simulink model "FCEvPowertrainController"  (R2024a)
settings: configuration reference "VehicleFixed10ms" (kept outside this file)
undefined symbols (not defined in the file): BattChrgMax, BattDischrgMax, ChrgLmt_bpt, CtrlBcuTrlrBrkGain, CtrlVcuEvChrgLmtBpt, CtrlVcuEvRegenBrkCutOff, CtrlVcuEvRegenBrkSpdBpt, CtrlVcuEvSocBpt, DischrgLmt_bpt, FCctrl, PlntBrkActrBoreFrnt, PlntBrkFrntBias, PlntBrkKinFricCffFrnt, PlntBrkNumPadsFrnt, PlntBrkPadMeanRadiusFrnt, PlntBrkPrsFctr, PlntBrkRearBias, PlntDiffrntlRatio, PlntEM1EffTbl, PlntEM1Spd, PlntEM1SpdEff, PlntEM1Trq, PlntEM1TrqEff, SOC_bpt
libraries: simulink x6, slpidlib x1, autolibutils x1
settings Model: DataDictionary=VirtualVehicleTemplate.sldd  ModifiedByFormat=The MathWorks, Inc.  SimulationMode=accelerator  Creator=The MathWorks, Inc.  LastModifiedBy=The MathWorks, Inc.
settings ConfigSetRef: SourceName=VehicleFixed10ms

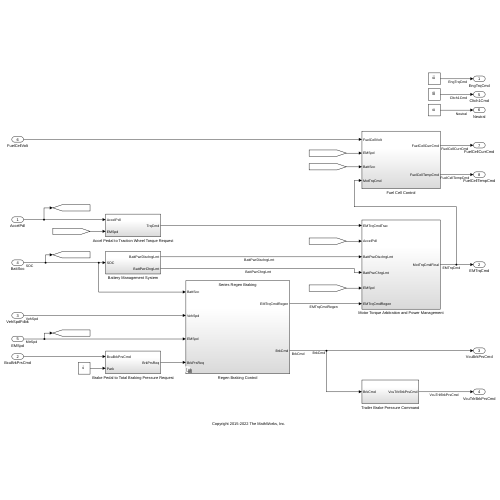
[thumbnail: Simulink's stored preview of the top-level diagram]
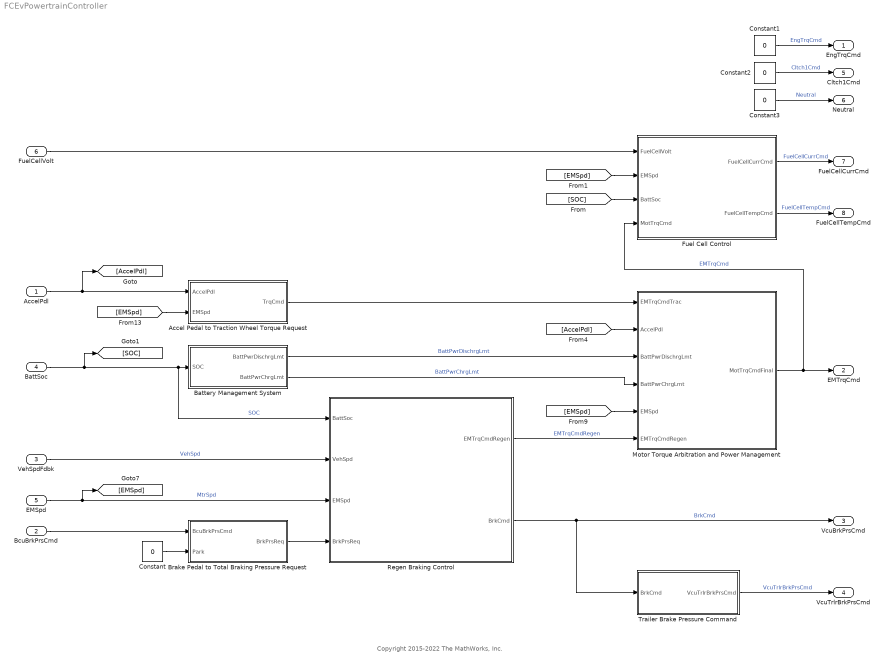
== system FCEvPowertrainController ==
  note: Copyright 2015-2022 The MathWorks, Inc.
  AccelPdl : Inport
  BcuBrkPrsCmd : Inport  Port=2  OutDataTypeStr=double  PortDimensions=4
  VehSpdFdbk : Inport  Port=3
  BattSoc : Inport  Port=4
  EMSpd : Inport  Port=5
  FuelCellVolt : Inport  Port=6
  Accel Pedal to Traction Wheel Torque Request : Subsystem  InitFcn=[~]=autosharedicon('autolibinternalvvblock',gcb,0);
  Battery Management System : Subsystem
  Brake Pedal to Total Braking Pressure Request : Subsystem
  Constant : Constant  Value=0
  Constant1 : Constant  Value=0  SampleTime=-1
  Constant2 : Constant  Value=0  SampleTime=-1
  Constant3 : Constant  Value=0  SampleTime=-1
  Fuel Cell Control : Subsystem
  Motor Torque Arbitration and Power Management : Subsystem
  Regen Braking Control : Subsystem  Variant=on  VariantControlMode=label  VariantControl=(default)  LabelModeActiveChoice=Variant
  Trailer Brake Pressure Command : Subsystem
  EngTrqCmd : Outport  OutDataTypeStr=double  PortDimensions=1  SampleTime=[0.01,0]  VectorParamsAs1DForOutWhenUnconnected=off
  EMTrqCmd : Outport  Port=2  VectorParamsAs1DForOutWhenUnconnected=off
  VcuBrkPrsCmd : Outport  Port=3  PortDimensions=4  VectorParamsAs1DForOutWhenUnconnected=off
  VcuTrlrBrkPrsCmd : Outport  Port=4  PortDimensions=6  VectorParamsAs1DForOutWhenUnconnected=off
  Cltch1Cmd : Outport  Port=5  PortDimensions=1  SampleTime=[0.01,0]  VectorParamsAs1DForOutWhenUnconnected=off
  Neutral : Outport  Port=6  PortDimensions=1  SampleTime=[0.01,0]  VectorParamsAs1DForOutWhenUnconnected=off
  FuelCellCurrCmd : Outport  Port=7  SampleTime=.01
  FuelCellTempCmd : Outport  Port=8
  wires:
  [AccelPdl] -> Motor Torque Arbitration and Power Management/2(AccelPdl)
  Battery Management System/1(BattPwrDischrgLmt) -> Motor Torque Arbitration and Power Management/3(BattPwrDischrgLmt)  "BattPwrDischrgLmt"
  BcuBrkPrsCmd/1 -> Brake Pedal to Total Braking Pressure Request/1(BcuBrkPrsCmd)
  Constant/1 -> Brake Pedal to Total Braking Pressure Request/2(Park)
  Battery Management System/2(BattPwrChrgLmt) -> Motor Torque Arbitration and Power Management/4("BattPwrChrgLmt ")  "BattPwrChrgLmt"
  Brake Pedal to Total Braking Pressure Request/1(BrkPrsReq) -> Regen Braking Control/4("BrkPrsReq ")
  [EMSpd] -> Accel Pedal to Traction Wheel Torque Request/2(EMSpd)
  VehSpdFdbk/1 -> Regen Braking Control/2("VehSpd ")  "VehSpd"
  BattSoc/1 -> [SOC], Regen Braking Control/1("BattSoc "), Battery Management System/1(SOC)  "SOC"
  Accel Pedal to Traction Wheel Torque Request/1(TrqCmd) -> Motor Torque Arbitration and Power Management/1(EMTrqCmdTrac)
  EMSpd/1 -> Regen Braking Control/3("EMSpd "), [EMSpd]  "MtrSpd"
  AccelPdl/1 -> [AccelPdl], Accel Pedal to Traction Wheel Torque Request/1(AccelPdl)
  [EMSpd] -> Motor Torque Arbitration and Power Management/5(EMSpd)
  Motor Torque Arbitration and Power Management/1(MotTrqCmdFinal) -> Fuel Cell Control/4(MotTrqCmd), EMTrqCmd/1  "EMTrqCmd"
  Regen Braking Control/1(" EMTrqCmdRegen") -> Motor Torque Arbitration and Power Management/6(EMTrqCmdRegen)  "EMTrqCmdRegen"
  FuelCellVolt/1 -> Fuel Cell Control/1(FuelCellVolt)
  [EMSpd] -> Fuel Cell Control/2(EMSpd)
  [SOC] -> Fuel Cell Control/3(BattSoc)
  Fuel Cell Control/1(FuelCellCurrCmd) -> FuelCellCurrCmd/1  "FuelCellCurrCmd"
  Fuel Cell Control/2(FuelCellTempCmd) -> FuelCellTempCmd/1  "FuelCellTempCmd"
  Constant3/1 -> Neutral/1  "Neutral"
  Constant2/1 -> Cltch1Cmd/1  "Cltch1Cmd"
  Constant1/1 -> EngTrqCmd/1  "EngTrqCmd"
  Trailer Brake Pressure Command/1(VcuTrlrBrkPrsCmd) -> VcuTrlrBrkPrsCmd/1  "VcuTrlrBrkPrsCmd"
  Regen Braking Control/2(" BrkCmd") -> Trailer Brake Pressure Command/1(BrkCmd), VcuBrkPrsCmd/1  "BrkCmd"

== system FCEvPowertrainController/Accel Pedal to Traction Wheel Torque Request ==
  note: Convert Accelerator Pedal Position to Torque Command
      | using Motor Torque Speed Curve
  AccelPdl : Inport
  EMSpd : Inport  Port=2
  MaxEMTrqVsSpd : Lookup_n-D  NumberOfTableDimensions=1  BreakpointsForDimension1=PlntEM1Spd  Table=PlntEM1Trq  ExtrapMethod=Clip  UseLastTableValue=on  InternalRulePriority=Speed  OutDataTypeStr=Inherit: Inherit from 'Table data'  RndMeth=Simplest
  Product1 : Product
  rads_to_rpm : Gain  Gain=30/pi
  TrqCmd : Outport  VectorParamsAs1DForOutWhenUnconnected=off
  wires:
  Product1/1 -> TrqCmd/1
  MaxEMTrqVsSpd/1 -> Product1/2
  AccelPdl/1 -> Product1/1
  EMSpd/1 -> rads_to_rpm/1
  rads_to_rpm/1 -> MaxEMTrqVsSpd/1

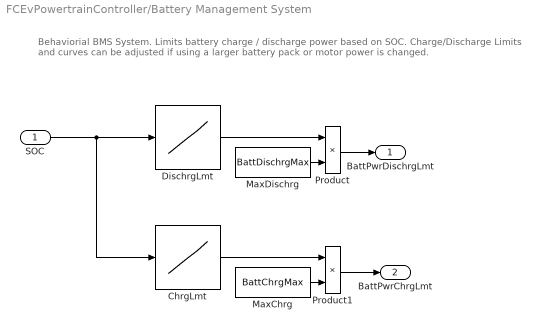
== system FCEvPowertrainController/Battery Management System ==
  note: Behaviorial BMS System. Limits battery charge / discharge power based on SOC.
      |
      | Charge/Discharge Limits and curves can be adjusted if using a larger battery pack
      | or motor power is changed.
  SOC : Inport
  ChrgLmt : Lookup_n-D  NumberOfTableDimensions=1  BreakpointsForDimension1=SOC_bpt  Table=ChrgLmt_bpt  ExtrapMethod=Clip  UseLastTableValue=on  InternalRulePriority=Speed  RndMeth=Simplest
  DischrgLmt : Lookup_n-D  NumberOfTableDimensions=1  BreakpointsForDimension1=SOC_bpt  Table=DischrgLmt_bpt  ExtrapMethod=Clip  UseLastTableValue=on  InternalRulePriority=Speed  RndMeth=Simplest
  MaxChrg : Constant  Value=BattChrgMax
  MaxDischrg : Constant  Value=BattDischrgMax
  Product : Product
  Product1 : Product
  BattPwrDischrgLmt : Outport  VectorParamsAs1DForOutWhenUnconnected=off
  BattPwrChrgLmt : Outport  Port=2  VectorParamsAs1DForOutWhenUnconnected=off
  wires:
  SOC/1 -> DischrgLmt/1, ChrgLmt/1
  MaxChrg/1 -> Product1/2
  MaxDischrg/1 -> Product/2
  Product/1 -> BattPwrDischrgLmt/1
  Product1/1 -> BattPwrChrgLmt/1
  ChrgLmt/1 -> Product1/1
  DischrgLmt/1 -> Product/1

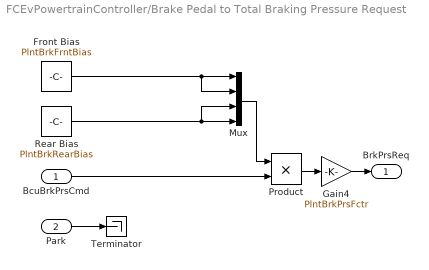
== system FCEvPowertrainController/Brake Pedal to Total Braking Pressure Request ==
  BcuBrkPrsCmd : Inport
  Park : Inport  Port=2
  Front Bias : Constant  Value=PlntBrkFrntBias
  Gain4 : Gain  Gain=PlntBrkPrsFctr
  Mux : Mux
  Product : Product
  Rear Bias : Constant  Value=PlntBrkRearBias
  Terminator : Terminator
  BrkPrsReq : Outport  VectorParamsAs1DForOutWhenUnconnected=off
  wires:
  BcuBrkPrsCmd/1 -> Product/2
  Mux/1 -> Product/1
  Rear Bias/1 -> Mux/4, Mux/3
  Front Bias/1 -> Mux/1, Mux/2
  Gain4/1 -> BrkPrsReq/1
  Product/1 -> Gain4/1
  Park/1 -> Terminator/1

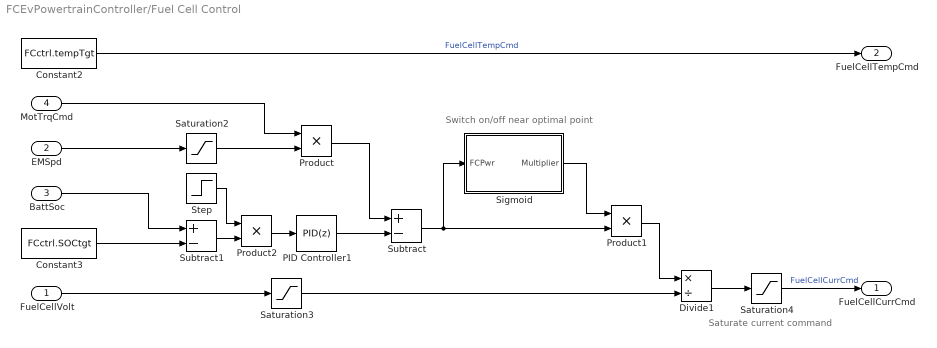
== system FCEvPowertrainController/Fuel Cell Control ==
  note: Switch on/off near optimal point
  note: Saturate current command
  FuelCellVolt : Inport
  EMSpd : Inport  Port=2
  BattSoc : Inport  Port=3
  MotTrqCmd : Inport  Port=4
  Constant2 : Constant  Value=FCctrl.tempTgt  SampleTime=0.01
  Constant3 : Constant  Value=FCctrl.SOCtgt
  Divide1 : Product  Inputs=*/
  PID Controller1 : slpidlib/PID Controller  Controller=PID  Form=Parallel  TimeDomain=Discrete-time  UseExternalTs=off  SampleTime=-1  IntegratorMethod=Forward Euler  FilterMethod=Forward Euler  ControllerParametersSource=internal  P=10000/2  I=0  UseKiTs=off  D=0  UseExternalDerivativeSource=off  N=100  UseFilter=on  TunerSelectOption=Transfer Function Based (PID Tuner App)  ZeroCross=off  InitialConditionSource=internal  InitialConditionForIntegrator=0  InitialConditionForFilter=0  DifferentiatorICPrevScaledInput=0  ExternalReset=none  TrackingMode=off  Kt=1  LimitOutput=off  SatLimitsSource=internal  UpperSaturationLimit=inf  LowerSaturationLimit=-inf  LinearizeAsGain=on  AntiWindupMode=none  Kb=1  LimitIntegrator=off  UpperIntegratorSaturationLimit=inf  LowerIntegratorSaturationLimit=-inf  POutMin=[]  POutMax=[]  IOutMin=[]  IOutMax=[]  DOutMin=[]  DOutMax=[]  NOutMin=[]  NOutMax=[]  SumOutMin=[]  SumOutMax=[]  SaturationOutMin=[]  SaturationOutMax=[]  PParamMin=[]  PParamMax=[]  IParamMin=[]  IParamMax=[]  DParamMin=[]  DParamMax=[]  NParamMin=[]  NParamMax=[]  KbParamMin=[]  KbParamMax=[]  KtParamMin=[]  KtParamMax=[]  KbOutMin=[]  KbOutMax=[]  KtOutMin=[]  KtOutMax=[]  IntegratorOutMin=[]  IntegratorOutMax=[]  FilterOutMin=[]  FilterOutMax=[]  SumI1OutMin=[]  SumI1OutMax=[]  SumI2OutMin=[]  SumI2OutMax=[]  SumI3OutMin=[]  SumI3OutMax=[]  SumI4OutMin=[]  SumI4OutMax=[]  SumDOutMin=[]  SumDOutMax=[]  DifferentiatorOutMin=[]  DifferentiatorOutMax=[]  FilterDiffOutCoefMin=[]  FilterDiffOutCoefMax=[]  ReciprocalOutMin=[]  ReciprocalOutMax=[]  SumDenOutMin=[]  SumDenOutMax=[]  SumNumOutMin=[]  SumNumOutMax=[]  DivideOutMin=[]  DivideOutMax=[]  UdiffTsProdOutMin=[]  UdiffTsProdOutMax=[]  NTsProdOutMin=[]  NTsProdOutMax=[]  UintegralTsProdOutMin=[]  UintegralTsProdOutMax=[]  UngainTsProdOutMin=[]  UngainTsProdOutMax=[]  ClampingZeroOutDataTypeStr=Inherit: Inherit via back propagation  ClampingZeroOutMin=[]  ClampingZeroOutMax=[]  FilterDenConstantOutDataTypeStr=Inherit: Inherit via back propagation  FilterDenConstantOutMin=[]  FilterDenConstantOutMax=[]  PCopyOutDataTypeStr=Inherit: Inherit via back propagation  PCopyOutMin=[]  PCopyOutMax=[]  NCopyOutDataTypeStr=Inherit: Inherit via back propagation  NCopyOutMin=[]  NCopyOutMax=[]  IntegratorContinuousStateAttributes=''  IntegratorStateMustResolveToSignalObject=off  IntegratorRTWStateStorageClass=Auto  FilterContinuousStateAttributes=''  FilterStateMustResolveToSignalObject=off  FilterRTWStateStorageClass=Auto  ParallelPVariant=InternalParameters  IdealPVariant=Disabled  IVariant=InternalParameters  DVariant=InternalParameters  IntegratorVariant=Discrete  SatVariant=Disabled  AWVariant=Passthrough  PCopyVariant=Disabled  TRVariant=Disabled  FdbkBlocksVariant=Forward  IdealPFdbkVariant=Disabled  SatFdbkVariant=Disabled  DerivativeFilterVariant=ForwardEulerFilter  NVariant=InternalParameters  NCopyVariant=Disabled  FilterICVariant=InternalICsFilter  IntegratorICVariant=InternalICs  ExternalResetVariant=Disabled  TRSumVariant=Passthrough  SumFdbkVariant=Disabled  SumVariant=Sum_PID  TsampFilterVariant=InternalTs  TsampNgainVariant=Passthrough  TsampIntegralVariant=Disabled_SignalSpec  ExternalSaturationOutDataTypeStr=Inherit: Same as second input  DerivativeSourceVariant=ErrorSignal
  Product : Product
  Product1 : Product
  Product2 : Product
  Saturation2 : Saturate  UpperLimit=inf  LowerLimit=1  ZeroCross=off
  Saturation3 : Saturate  UpperLimit=inf  LowerLimit=200  ZeroCross=off
  Saturation4 : Saturate  UpperLimit=350  LowerLimit=0  ZeroCross=off
  Sigmoid : Subsystem
  Step : Step  SampleTime=0.01
  Subtract : Sum  Inputs=+-
  Subtract1 : Sum  Inputs=+-
  FuelCellCurrCmd : Outport  SampleTime=.01
  FuelCellTempCmd : Outport  Port=2
  wires:
  MotTrqCmd/1 -> Product/1
  Saturation4/1 -> FuelCellCurrCmd/1  "FuelCellCurrCmd"
  PID Controller1/1 -> Subtract/2
  Sigmoid/1(Multiplier) -> Product1/1
  Divide1/1 -> Saturation4/1
  Saturation3/1 -> Divide1/2
  Subtract/1 -> Product1/2, Sigmoid/1(FCPwr)
  Product/1 -> Subtract/1
  EMSpd/1 -> Saturation2/1
  Saturation2/1 -> Product/2
  BattSoc/1 -> Subtract1/1
  FuelCellVolt/1 -> Saturation3/1
  Product1/1 -> Divide1/1
  Constant3/1 -> Subtract1/2
  Constant2/1 -> FuelCellTempCmd/1  "FuelCellTempCmd"
  Subtract1/1 -> Product2/2
  Product2/1 -> PID Controller1/1
  Step/1 -> Product2/1

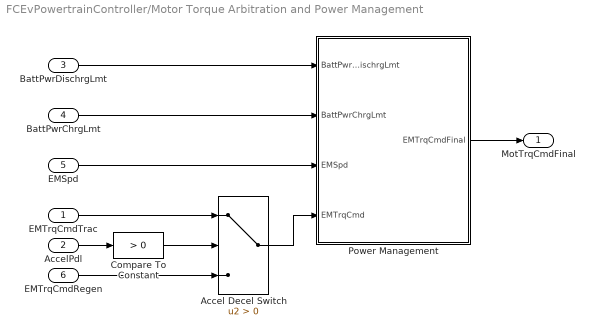
== system FCEvPowertrainController/Motor Torque Arbitration and Power Management ==
  EMTrqCmdTrac : Inport
  AccelPdl : Inport  Port=2
  BattPwrDischrgLmt : Inport  Port=3
  "BattPwrChrgLmt " : Inport  Port=4
  EMSpd : Inport  Port=5
  EMTrqCmdRegen : Inport  Port=6
  Accel Decel Switch : Switch  Criteria=u2 > Threshold  SaturateOnIntegerOverflow=off  InputSameDT=off
  Compare To Constant : simulink/Logic and Bit Operations/Compare To Constant  relop=>  const=0  OutDataTypeStr=boolean
  Power Management : Subsystem
  MotTrqCmdFinal : Outport  VectorParamsAs1DForOutWhenUnconnected=off
  wires:
  AccelPdl/1 -> Compare To Constant/1
  EMTrqCmdRegen/1 -> Accel Decel Switch/3
  EMTrqCmdTrac/1 -> Accel Decel Switch/1
  Power Management/1(EMTrqCmdFinal) -> MotTrqCmdFinal/1
  Accel Decel Switch/1 -> Power Management/4(EMTrqCmd)
  BattPwrDischrgLmt/1 -> Power Management/1(BattPwrDischrgLmt)
  "BattPwrChrgLmt "/1 -> Power Management/2(BattPwrChrgLmt)
  EMSpd/1 -> Power Management/3(EMSpd)
  Compare To Constant/1 -> Accel Decel Switch/2

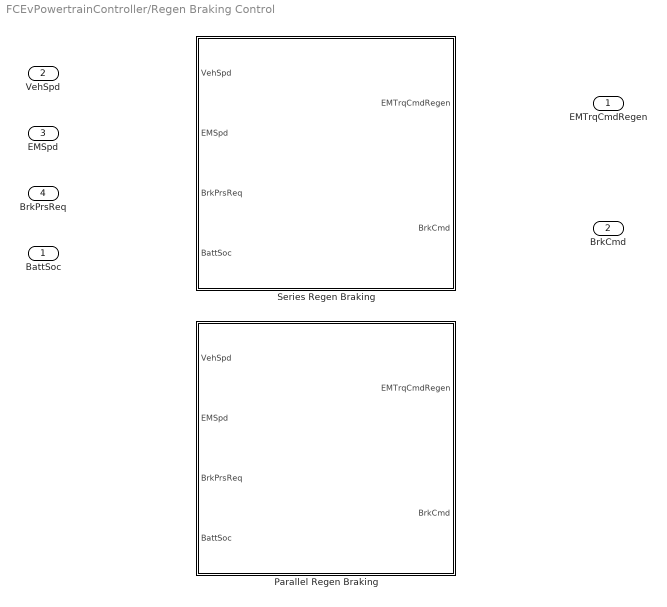
== system FCEvPowertrainController/Regen Braking Control ==
  "BattSoc " : Inport
  "VehSpd " : Inport  Port=2
  "EMSpd " : Inport  Port=3
  "BrkPrsReq " : Inport  Port=4
  Parallel Regen Braking : Subsystem  InitFcn=[~]=autosharedicon('autolibinternalvvblock',gcb,0);  VariantControl=(default)
  Series Regen Braking : Subsystem  InitFcn=[~]=autosharedicon('autolibinternalvvblock',gcb,0);  VariantControl=Variant
  " EMTrqCmdRegen" : Outport  VectorParamsAs1DForOutWhenUnconnected=off
  " BrkCmd" : Outport  Port=2  VectorParamsAs1DForOutWhenUnconnected=off

== system FCEvPowertrainController/Trailer Brake Pressure Command ==
  BrkCmd : Inport
  Gain1 : Gain  Gain=CtrlBcuTrlrBrkGain
  Probe : Probe  ProbeSampleTime=off  ProbeComplexSignal=off
  Product : Product  Inputs=*/
  Selector2 : Selector  InputPortWidth=1  IndexOptions=Index vector (dialog)  Indices=[1 1 1 1 1 1]  OutputSizes=1
  Sum : Sum  Inputs=+
  VcuTrlrBrkPrsCmd : Outport
  wires:
  Gain1/1 -> Selector2/1
  Product/1 -> Gain1/1
  Probe/1 -> Product/2
  BrkCmd/1 -> Probe/1, Sum/1
  Sum/1 -> Product/1
  Selector2/1 -> VcuTrlrBrkPrsCmd/1

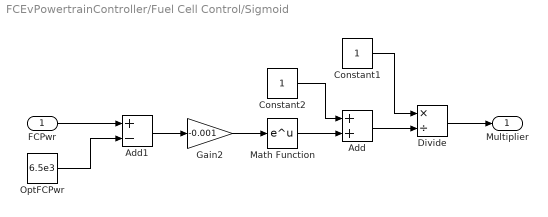
== system FCEvPowertrainController/Fuel Cell Control/Sigmoid ==
  FCPwr : Inport
  Add : Sum
  Add1 : Sum  Inputs=+-
  Constant1 : Constant
  Constant2 : Constant
  Divide : Product  Inputs=*/
  Gain2 : Gain  Gain=-0.001
  Math Function : Math
  OptFCPwr : Constant  Value=6.5e3
  Multiplier : Outport
  wires:
  Add1/1 -> Gain2/1
  Divide/1 -> Multiplier/1
  Math Function/1 -> Add/2
  Add/1 -> Divide/2
  OptFCPwr/1 -> Add1/2
  Constant2/1 -> Add/1
  FCPwr/1 -> Add1/1
  Gain2/1 -> Math Function/1
  Constant1/1 -> Divide/1

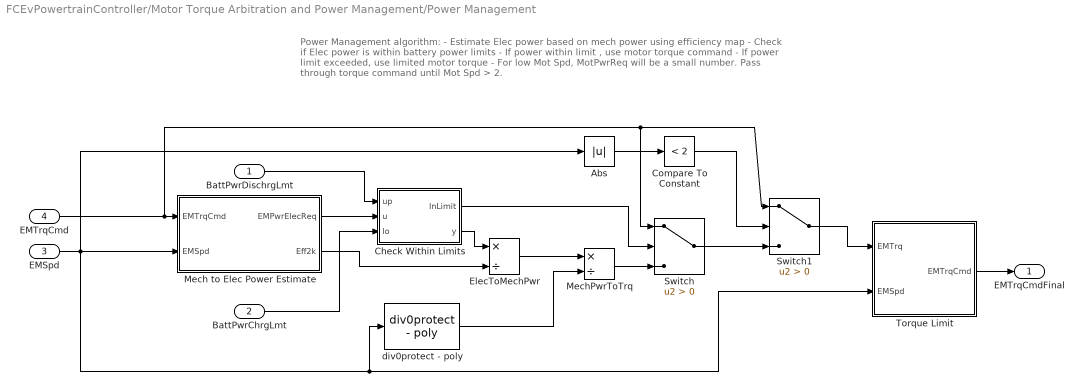
== system FCEvPowertrainController/Motor Torque Arbitration and Power Management/Power Management ==
  note: Power Management algorithm:
      | - Estimate Elec power based on mech power using efficiency map
      | - Check if Elec power is within battery power limits
      | - If power within limit , use motor torque command
      | - If power limit exceeded, use limited motor torque
      | - For low Mot Spd, MotPwrReq will be a small number.  Pass through torque command until Mot Spd > 2.
  BattPwrDischrgLmt : Inport
  BattPwrChrgLmt : Inport  Port=2
  EMSpd : Inport  Port=3
  EMTrqCmd : Inport  Port=4
  Abs : Abs  SaturateOnIntegerOverflow=off
  Check Within Limits : Subsystem
  Compare To Constant : simulink/Logic and Bit Operations/Compare To Constant  relop=<  const=2  OutDataTypeStr=boolean
  ElecToMechPwr : Product  Inputs=*/
  Mech to Elec Power Estimate : Subsystem
  MechPwrToTrq : Product  Inputs=*/
  Switch : Switch  Criteria=u2 > Threshold  SaturateOnIntegerOverflow=off  InputSameDT=off
  Switch1 : Switch  Criteria=u2 > Threshold  SaturateOnIntegerOverflow=off  InputSameDT=off
  Torque Limit : Subsystem
  div0protect - poly : autolibutils/div0protect - poly  thresh=2  ZeroCross1=off  aMode=aMode
  EMTrqCmdFinal : Outport  VectorParamsAs1DForOutWhenUnconnected=off
  wires:
  EMSpd/1 -> Abs/1, Torque Limit/2(EMSpd), div0protect - poly/1, Mech to Elec Power Estimate/2(EMSpd)
  EMTrqCmd/1 -> Switch/1, Switch1/1, Mech to Elec Power Estimate/1(EMTrqCmd)
  div0protect - poly/1 -> MechPwrToTrq/2
  Mech to Elec Power Estimate/2(Eff2k) -> ElecToMechPwr/2
  ElecToMechPwr/1 -> MechPwrToTrq/1
  MechPwrToTrq/1 -> Switch/3
  Torque Limit/1(EMTrqCmd) -> EMTrqCmdFinal/1
  BattPwrDischrgLmt/1 -> Check Within Limits/1(up)
  Mech to Elec Power Estimate/1(EMPwrElecReq) -> Check Within Limits/2(u)
  BattPwrChrgLmt/1 -> Check Within Limits/3(lo)
  Check Within Limits/2(y) -> ElecToMechPwr/1
  Switch/1 -> Switch1/3
  Check Within Limits/1(InLimit) -> Switch/2
  Switch1/1 -> Torque Limit/1(EMTrq)
  Abs/1 -> Compare To Constant/1
  Compare To Constant/1 -> Switch1/2

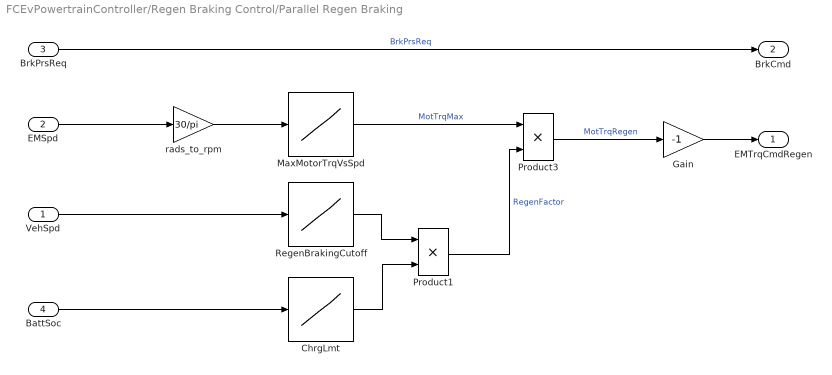
== system FCEvPowertrainController/Regen Braking Control/Parallel Regen Braking ==
  VehSpd : Inport
  "EMSpd " : Inport  Port=2
  "BrkPrsReq " : Inport  Port=3
  BattSoc : Inport  Port=4
  ChrgLmt : Lookup_n-D  NumberOfTableDimensions=1  BreakpointsForDimension1=CtrlVcuEvSocBpt  Table=CtrlVcuEvChrgLmtBpt  ExtrapMethod=Clip  UseLastTableValue=on  InternalRulePriority=Speed  RndMeth=Simplest
  Gain : Gain  Gain=-1
  MaxMotorTrqVsSpd : Lookup_n-D  NumberOfTableDimensions=1  BreakpointsForDimension1=PlntEM1Spd*30/pi  Table=PlntEM1Trq  ExtrapMethod=Clip  UseLastTableValue=on  InternalRulePriority=Speed  OutDataTypeStr=Inherit: Inherit from 'Table data'  RndMeth=Simplest
  Product1 : Product
  Product3 : Product
  RegenBrakingCutoff : Lookup_n-D  NumberOfTableDimensions=1  BreakpointsForDimension1=CtrlVcuEvRegenBrkSpdBpt  Table=CtrlVcuEvRegenBrkCutOff  ExtrapMethod=Clip  UseLastTableValue=on  InternalRulePriority=Speed  RndMeth=Simplest
  rads_to_rpm : Gain  Gain=30/pi
  " EMTrqCmdRegen" : Outport  VectorParamsAs1DForOutWhenUnconnected=off
  " BrkCmd" : Outport  Port=2  VectorParamsAs1DForOutWhenUnconnected=off
  wires:
  Gain/1 -> " EMTrqCmdRegen"/1
  BattSoc/1 -> ChrgLmt/1
  Product3/1 -> Gain/1  "MotTrqRegen"
  Product1/1 -> Product3/2  "RegenFactor"
  RegenBrakingCutoff/1 -> Product1/1
  VehSpd/1 -> RegenBrakingCutoff/1
  ChrgLmt/1 -> Product1/2
  MaxMotorTrqVsSpd/1 -> Product3/1  "MotTrqMax"
  rads_to_rpm/1 -> MaxMotorTrqVsSpd/1
  "EMSpd "/1 -> rads_to_rpm/1
  "BrkPrsReq "/1 -> " BrkCmd"/1  "BrkPrsReq"

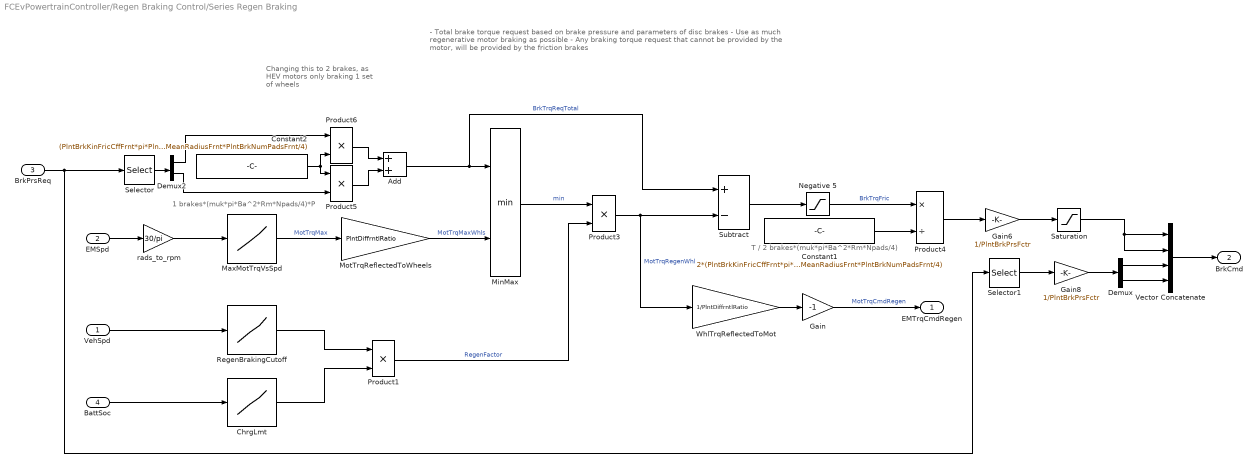
== system FCEvPowertrainController/Regen Braking Control/Series Regen Braking ==
  note: - Total brake torque request based on brake pressure and parameters of disc brakes
      | - Use as much regenerative motor braking as possible
      | - Any braking torque request that cannot be provided by the motor, will be provided by the friction brakes
  note: T / 2 brakes*(muk*pi*Ba^2*Rm*Npads/4)
  note: Changing this to 2 brakes,
      | as HEV motors only braking
      | 1 set of wheels
  note: 1 brakes*(muk*pi*Ba^2*Rm*Npads/4)*P
  VehSpd : Inport
  "EMSpd " : Inport  Port=2
  "BrkPrsReq " : Inport  Port=3
  BattSoc : Inport  Port=4
  Add : Sum
  ChrgLmt : Lookup_n-D  NumberOfTableDimensions=1  BreakpointsForDimension1=CtrlVcuEvSocBpt  Table=CtrlVcuEvChrgLmtBpt  ExtrapMethod=Clip  UseLastTableValue=on  InternalRulePriority=Speed  RndMeth=Simplest
  Constant1 : Constant  Value=2*(PlntBrkKinFricCffFrnt*pi*PlntBrkActrBoreFrnt^2*PlntBrkPadMeanRadiusFrnt*PlntBrkNumPadsFrnt/4)
  Constant2 : Constant  Value=(PlntBrkKinFricCffFrnt*pi*PlntBrkActrBoreFrnt^2*PlntBrkPadMeanRadiusFrnt*PlntBrkNumPadsFrnt/4)
  Demux : Demux  Outputs=2
  Demux2 : Demux  Outputs=2
  Gain : Gain  Gain=-1
  Gain6 : Gain  Gain=1/PlntBrkPrsFctr
  Gain8 : Gain  Gain=1/PlntBrkPrsFctr
  MaxMotTrqVsSpd : Lookup_n-D  NumberOfTableDimensions=1  BreakpointsForDimension1=PlntEM1Spd*30/pi  Table=PlntEM1Trq  ExtrapMethod=Clip  UseLastTableValue=on  InternalRulePriority=Speed  OutDataTypeStr=Inherit: Inherit from 'Table data'  RndMeth=Simplest
  MinMax : MinMax  Inputs=2
  MotTrqReflectedToWheels : Gain  Gain=PlntDiffrntlRatio
  Negative 5 : Saturate  UpperLimit=inf  LowerLimit=0
  Product{1,3,5..6} (4 alike) : Product
  Product4 : Product  Inputs=*/
  RegenBrakingCutoff : Lookup_n-D  NumberOfTableDimensions=1  BreakpointsForDimension1=CtrlVcuEvRegenBrkSpdBpt  Table=CtrlVcuEvRegenBrkCutOff  ExtrapMethod=Clip  UseLastTableValue=on  InternalRulePriority=Speed  RndMeth=Simplest
  Saturation : Saturate  UpperLimit=1  LowerLimit=0
  Selector : Selector  InputPortWidth=4  IndexOptions=Index vector (dialog)  Indices=[1 2]  OutputSizes=1
  Selector1 : Selector  InputPortWidth=4  IndexOptions=Index vector (dialog)  Indices=[3 4]  OutputSizes=1
  Subtract : Sum  Inputs=+-
  Vector Concatenate : Concatenate  NumInputs=4
  WhlTrqReflectedToMot : Gain  Gain=1/PlntDiffrntlRatio
  rads_to_rpm : Gain  Gain=30/pi
  " EMTrqCmdRegen" : Outport  VectorParamsAs1DForOutWhenUnconnected=off
  " BrkCmd" : Outport  Port=2  VectorParamsAs1DForOutWhenUnconnected=off
  wires:
  Product3/1 -> WhlTrqReflectedToMot/1, Subtract/2  "MotTrqRegenWhl"
  Constant1/1 -> Product4/2
  rads_to_rpm/1 -> MaxMotTrqVsSpd/1
  MaxMotTrqVsSpd/1 -> MotTrqReflectedToWheels/1  "MotTrqMax"
  MinMax/1 -> Product3/1  "min"
  ChrgLmt/1 -> Product1/2
  VehSpd/1 -> RegenBrakingCutoff/1
  RegenBrakingCutoff/1 -> Product1/1
  Product1/1 -> Product3/2  "RegenFactor"
  Subtract/1 -> Negative 5/1
  BattSoc/1 -> ChrgLmt/1
  Negative 5/1 -> Product4/1  "BrkTrqFric"
  "EMSpd "/1 -> rads_to_rpm/1
  MotTrqReflectedToWheels/1 -> MinMax/2  "MotTrqMaxWhls"
  WhlTrqReflectedToMot/1 -> Gain/1
  Gain/1 -> " EMTrqCmdRegen"/1  "MotTrqCmdRegen"
  Demux2/2 -> Product5/2
  Constant2/1 -> Product6/2, Product5/1
  Demux2/1 -> Product6/1
  Selector/1 -> Demux2/1
  Product6/1 -> Add/1
  Product5/1 -> Add/2
  Add/1 -> Subtract/1, MinMax/1  "BrkTrqReqTotal"
  Gain8/1 -> Demux/1
  Saturation/1 -> Vector Concatenate/2, Vector Concatenate/1
  Selector1/1 -> Gain8/1
  "BrkPrsReq "/1 -> Selector1/1, Selector/1
  Vector Concatenate/1 -> " BrkCmd"/1
  Gain6/1 -> Saturation/1
  Demux/1 -> Vector Concatenate/3
  Product4/1 -> Gain6/1
  Demux/2 -> Vector Concatenate/4

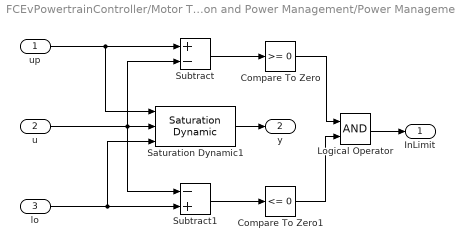
== system FCEvPowertrainController/Motor Torque Arbitration and Power Management/Power Management/Check Within Limits ==
  up : Inport
  u : Inport  Port=2
  lo : Inport  Port=3
  Compare To Zero : simulink/Logic and Bit Operations/Compare To Zero  relop=>=  OutDataTypeStr=boolean
  Compare To Zero1 : simulink/Logic and Bit Operations/Compare To Zero  relop=<=  OutDataTypeStr=boolean
  Logical Operator : Logic  AllPortsSameDT=off  OutDataTypeStr=boolean
  Saturation Dynamic1 : simulink/Discontinuities/Saturation Dynamic  OutMin=[]  OutMax=[]  OutDataTypeStr=Inherit: Same as second input  OutDataType=fixdt(1, 16)  OutScaling=2^-10  DoSatur=off
  Subtract : Sum  Inputs=+-
  Subtract1 : Sum  Inputs=-+
  InLimit : Outport  VectorParamsAs1DForOutWhenUnconnected=off
  y : Outport  Port=2  VectorParamsAs1DForOutWhenUnconnected=off
  wires:
  Saturation Dynamic1/1 -> y/1
  lo/1 -> Subtract1/2, Saturation Dynamic1/3
  up/1 -> Subtract/1, Saturation Dynamic1/1
  u/1 -> Subtract1/1, Subtract/2, Saturation Dynamic1/2
  Subtract/1 -> Compare To Zero/1
  Subtract1/1 -> Compare To Zero1/1
  Compare To Zero/1 -> Logical Operator/1
  Compare To Zero1/1 -> Logical Operator/2
  Logical Operator/1 -> InLimit/1

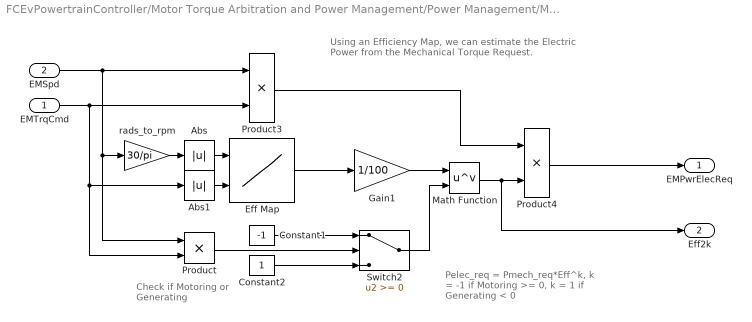
== system FCEvPowertrainController/Motor Torque Arbitration and Power Management/Power Management/Mech to Elec Power Estimate ==
  note: Check if Motoring
      | or Generating
  note: Using an Efficiency Map, we can estimate the
      | Electric Power from the Mechanical  Torque Request.
  note: Pelec_req = Pmech_req*Eff^k,
      | k = -1 if Motoring >= 0,
      | k = 1 if Generating < 0
  EMTrqCmd : Inport
  EMSpd : Inport  Port=2
  Abs : Abs  SaturateOnIntegerOverflow=off
  Abs1 : Abs  SaturateOnIntegerOverflow=off
  Constant1 : Constant  Value=-1  SampleTime=-1
  Constant2 : Constant  SampleTime=-1
  Eff Map : Lookup_n-D  BreakpointsForDimension1=PlntEM1SpdEff  BreakpointsForDimension2=PlntEM1TrqEff  Table=PlntEM1EffTbl  ExtrapMethod=Clip  UseLastTableValue=on  InternalRulePriority=Speed  OutDataTypeStr=Inherit: Inherit from 'Table data'  RndMeth=Simplest
      settings: InputPortMap=u0,u1
  Gain1 : Gain  Gain=1/100
  Math Function : Math  Operator=pow  SignedPower=on  OutputSignalType=real
  Product : Product
  Product3 : Product
  Product4 : Product
  Switch2 : Switch  SaturateOnIntegerOverflow=off  InputSameDT=off
  rads_to_rpm : Gain  Gain=30/pi
  EMPwrElecReq : Outport  VectorParamsAs1DForOutWhenUnconnected=off
  Eff2k : Outport  Port=2  VectorParamsAs1DForOutWhenUnconnected=off
  wires:
  Product3/1 -> Product4/1
  Switch2/1 -> Math Function/2
  Constant1/1 -> Switch2/1
  Constant2/1 -> Switch2/3
  Eff Map/1 -> Gain1/1
  Abs/1 -> Eff Map/1
  Gain1/1 -> Math Function/1
  Math Function/1 -> Eff2k/1, Product4/2
  Product4/1 -> EMPwrElecReq/1
  Abs1/1 -> Eff Map/2
  rads_to_rpm/1 -> Abs/1
  Product/1 -> Switch2/2
  EMSpd/1 -> Product3/1, Product/1, rads_to_rpm/1
  EMTrqCmd/1 -> Product3/2, Product/2, Abs1/1

== system FCEvPowertrainController/Motor Torque Arbitration and Power Management/Power Management/Torque Limit ==
  EMTrq : Inport
  EMSpd : Inport  Port=2
  Gain : Gain  Gain=-1
  MaxEMTrqVsSpd : Lookup_n-D  NumberOfTableDimensions=1  BreakpointsForDimension1=PlntEM1Spd  Table=PlntEM1Trq  ExtrapMethod=Clip  UseLastTableValue=on  InternalRulePriority=Speed  OutDataTypeStr=Inherit: Inherit from 'Table data'  RndMeth=Simplest
  Saturation Dynamic : simulink/Discontinuities/Saturation Dynamic  OutMin=[]  OutMax=[]  OutDataTypeStr=Inherit: Same as second input  OutDataType=fixdt(1, 16)  OutScaling=2^-10  DoSatur=off
  rads_to_rpm : Gain  Gain=30/pi
  EMTrqCmd : Outport  VectorParamsAs1DForOutWhenUnconnected=off
  wires:
  EMTrq/1 -> Saturation Dynamic/2
  Saturation Dynamic/1 -> EMTrqCmd/1
  EMSpd/1 -> rads_to_rpm/1
  MaxEMTrqVsSpd/1 -> Gain/1, Saturation Dynamic/1
  rads_to_rpm/1 -> MaxEMTrqVsSpd/1
  Gain/1 -> Saturation Dynamic/3
